simulink model "p2_linearWindTurbineModel"  (R2016b)
settings: Solver=ode4  StartTime=0.0  StopTime=TIME_SIM  FixedStep=STEP_SIZE  RelTol=1e-3
values from neighbouring files (symbols this model uses):
  Ts = 0.05    [relevantWindTurbineParameters.mat]
undefined symbols (not defined in the file or in its folder): Aa, Bb, Bv, Cc, K_FSF, Ki, xOP
settings Model: Creator=Aleks  LastModifiedBy=Fabio Spagnolo

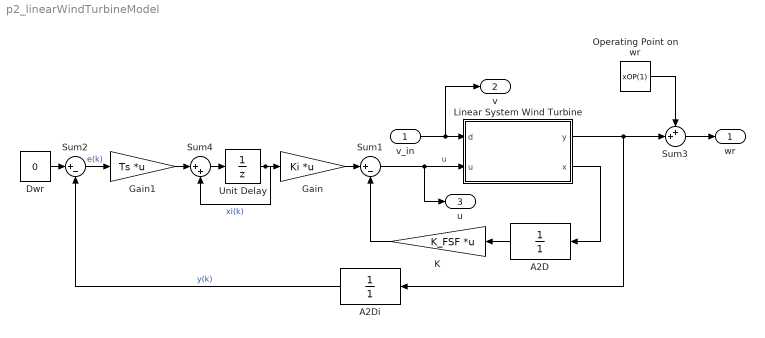
== system p2_linearWindTurbineModel ==
  v_in : Inport
  A2D : DiscreteTransferFcn  Denominator=[1]  SampleTime=Ts
  A2Di : DiscreteTransferFcn  Denominator=[1]  SampleTime=Ts
  Dwr : Constant  Value=0  SampleTime=Ts
  Gain : Gain  Gain=Ki  Multiplication=Matrix(K*u) (u vector)
  Gain1 : Gain  Gain=Ts  Multiplication=Matrix(K*u) (u vector)
  K : Gain  Gain=K_FSF  Multiplication=Matrix(K*u) (u vector)
  Linear System Wind Turbine : Subsystem
  Operating Point on wr : Constant  Value=xOP(1)
  Sum1 : Sum  Inputs=|+-
  Sum2 : Sum  Inputs=|+-
  Sum3 : Sum  Inputs=++|
  Sum4 : Sum  Inputs=|++
  Unit Delay : UnitDelay  SampleTime=Ts
  wr : Outport
  v : Outport  Port=2
  u : Outport  Port=3
  wires:
  Unit Delay/1 -> Gain/1, Sum4/2  "xi(k)"
  A2Di/1 -> Sum2/2  "y(k)"
  K/1 -> Sum1/2
  Sum3/1 -> wr/1
  A2D/1 -> K/1
  Sum4/1 -> Unit Delay/1
  Operating Point on wr/1 -> Sum3/1
  Gain/1 -> Sum1/1
  Dwr/1 -> Sum2/1
  Sum2/1 -> Gain1/1  "e(k)"
  Gain1/1 -> Sum4/1
  Linear System Wind Turbine/1(y) -> Sum3/2, A2Di/1
  v_in/1 -> v/1, Linear System Wind Turbine/1(d)
  Sum1/1 -> u/1, Linear System Wind Turbine/2(u)  "u"
  Linear System Wind Turbine/2(x) -> A2D/1

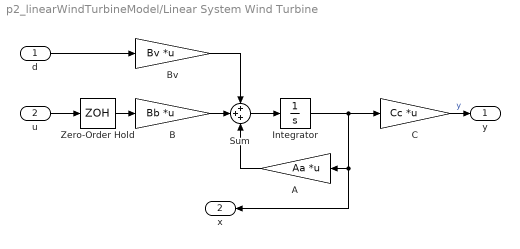
== system p2_linearWindTurbineModel/Linear System Wind Turbine ==
  d : Inport
  u : Inport  Port=2
  A : Gain  Gain=Aa  Multiplication=Matrix(K*u) (u vector)
  B : Gain  Gain=Bb  Multiplication=Matrix(K*u) (u vector)
  Bv : Gain  Gain=Bv  Multiplication=Matrix(K*u) (u vector)
  C : Gain  Gain=Cc  Multiplication=Matrix(K*u) (u vector)
  Integrator : Integrator
  Sum : Sum  Inputs=+++
  Zero-Order Hold : ZeroOrderHold  SampleTime=Ts
  y : Outport
  x : Outport  Port=2
  wires:
  Bv/1 -> Sum/1
  Sum/1 -> Integrator/1
  Integrator/1 -> A/1, x/1, C/1
  u/1 -> Zero-Order Hold/1
  A/1 -> Sum/3
  Zero-Order Hold/1 -> B/1
  B/1 -> Sum/2
  C/1 -> y/1  "y"
  d/1 -> Bv/1
